simulink model "Model"  (R2017a)
settings: Solver=FixedStepDiscrete  StartTime=0.0  StopTime=10.0  RelTol=1e-3
libraries: c2000scilib x1
settings Model: DataTypeOverride=Off  Creator=Aba  LastModifiedBy=Aba
settings DataIOCC: SaveOutput=off  SaveTime=off
settings OptimizationCC: BlockReduction=off  ConditionallyExecuteInputs=off  DefaultParameterBehavior=Inlined
settings DebuggingCC: AlgebraicLoopMsg=error  SingleTaskRateTransMsg=error  StrictBusMsg=ErrorOnBusTreatedAsVector
settings HardwareCC: ProdBitPerPointer=32  ProdBitPerSizeT=32  ProdBitPerPtrDiffT=32  ProdLargestAtomicFloat=None  ProdIntDivRoundTo=Undefined  ProdEndianess=Unspecified  ProdWordSize=32  ProdHWDeviceType=ASIC/FPGA->ASIC/FPGA  ProdEqTarget=off
settings GRTTargetCC: TargetLangStandard=C89/C90 (ANSI)

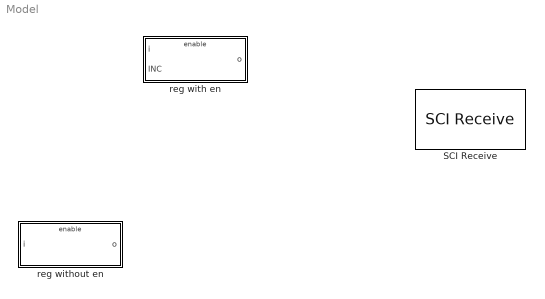
== system Model ==
  SCI Receive : c2000scilib/SCI Receive  module=COM 1  dataHead='S'  dataTail='E'  dataType=uint8  dataDim=1  initValue=0  errOption=Output the last received value  errValue=0  sampleTime=-1  outputStatus=off
  reg with en : Subsystem  TreatAsAtomicUnit=on
  reg without en : Subsystem  TreatAsAtomicUnit=on

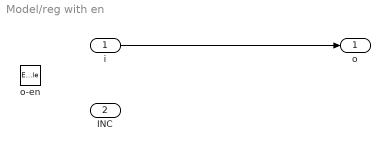
== system Model/reg with en ==
  i : Inport
  INC : Inport  Port=2
  o-en : EnablePort
  o : Outport
  wires:
  i/1 -> o/1

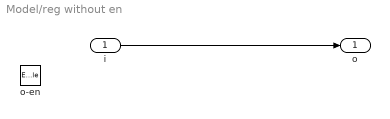
== system Model/reg without en ==
  i : Inport
  o-en : EnablePort
  o : Outport
  wires:
  i/1 -> o/1
